simulink model "DoublePendulum"  (R2015a)
settings: Solver=ode45  StartTime=0.0  StopTime=10  RelTol=1e-3
values from neighbouring files (symbols this model uses):
  g = 9.8    [DoublePendulum_config.m]
  J1 = 1.0    (= 1)    [DoublePendulum_config.m]
  J2 = 1.0    (= 1)    [DoublePendulum_config.m]
  l1 = 2.0    (= 2)    [DoublePendulum_config.m]
  l2 = 1.0    (= 1)    [DoublePendulum_config.m]
  lg1 = 1.2    [DoublePendulum_config.m]
  lg2 = 0.5    [DoublePendulum_config.m]
  m1 = 1.0    (= 1)    [DoublePendulum_config.m]
  m2 = 1.0    (= 1)    [DoublePendulum_config.m]
settings Model: Creator=hamada  LastModifiedBy=hamada

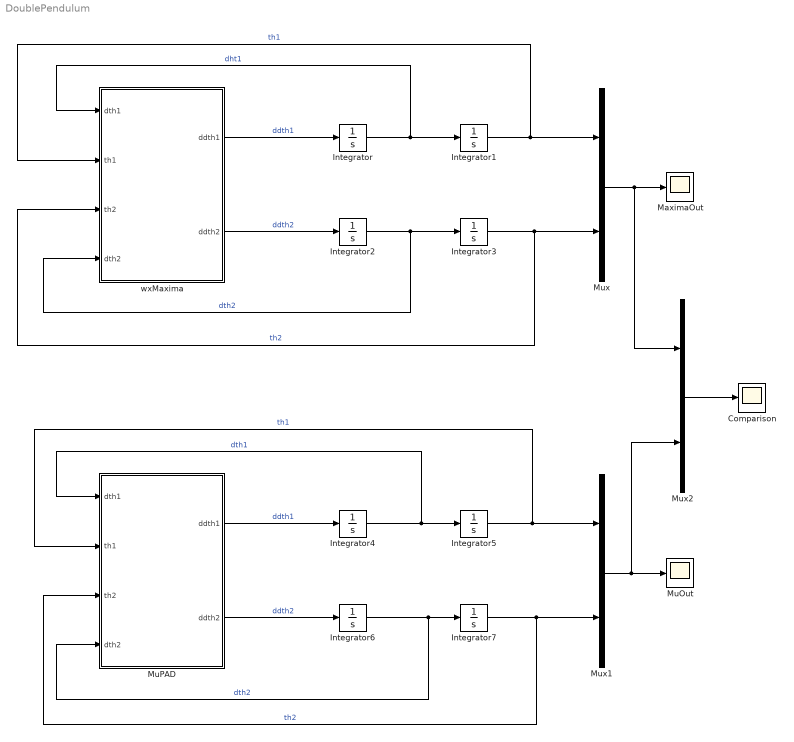
== system DoublePendulum ==
  Comparison : Scope
      settings: TimeRange=10  YMax=15  SaveName=MaximaOut1  SampleInput=on  SampleTime=0.1
  Integrator{,2..4,6..7} (6 alike) : Integrator
  Integrator1 : Integrator  InitialCondition=pi/2
  Integrator5 : Integrator  InitialCondition=pi/2
  MaximaOut : Scope
      settings: TimeRange=10  YMax=15  SaveName=MaximaOut  SampleInput=on  SampleTime=0.1
  MuOut : Scope
      settings: SaveName=MuOut  SampleInput=on  SampleTime=0.1
  MuPAD : MATLAB Function  TreatAsAtomicUnit=on
  Mux : Mux  Inputs=2
  Mux1 : Mux  Inputs=2
  Mux2 : Mux  Inputs=2
  wxMaxima : MATLAB Function  TreatAsAtomicUnit=on
  wires:
  wxMaxima/1(ddth1) -> Integrator/1  "ddth1"
  Integrator/1 -> wxMaxima/1(dth1), Integrator1/1  "dht1"
  Integrator1/1 -> Mux/1, wxMaxima/2(th1)  "th1"
  wxMaxima/2(ddth2) -> Integrator2/1  "ddth2"
  Integrator2/1 -> wxMaxima/4(dth2), Integrator3/1  "dth2"
  Integrator3/1 -> Mux/2, wxMaxima/3(th2)  "th2"
  Mux/1 -> Mux2/1, MaximaOut/1
  MuPAD/1(ddth1) -> Integrator4/1  "ddth1"
  MuPAD/2(ddth2) -> Integrator6/1  "ddth2"
  Integrator4/1 -> MuPAD/1(dth1), Integrator5/1  "dth1"
  Integrator6/1 -> MuPAD/4(dth2), Integrator7/1  "dth2"
  Integrator5/1 -> Mux1/1, MuPAD/2(th1)  "th1"
  Integrator7/1 -> Mux1/2, MuPAD/3(th2)  "th2"
  Mux1/1 -> Mux2/2, MuOut/1
  Mux2/1 -> Comparison/1

== matlab function DoublePendulum/MuPAD ==
  data: dth1 input double size=1; ddth1 output double size=1; th1 input double size=1; th2 input double size=1; dth2 input double size=1; lg1 parameter double size=1; l1 parameter double size=1; lg2 parameter double size=1; l2 parameter double size=1; m1 parameter double size=1; m2 parameter double size=1; J1 parameter double size=1; J2 parameter double size=1; ddth2 output double size=1; g parameter double size=1
function [ ddth1, ddth2 ] = fcn( dth1, th1, th2, dth2, lg1, l1, lg2, l2, m1, m2, J1, J2, g )
    %#codegen
    ddth1 = (sin(th2*2.0)*dth1^2*l1^2*lg2^2*m2^2+g*sin(th1)*l1*lg2^2*m2^2-g*sin(th1+th2*2.0)*l1*lg2^2*m2^2+sin(th2)*dth1^2*l1*lg2^3*m2^2*2.0+sin(th2)*dth2^2*l1*lg2^3*m2^2*2.0+g*sin(th1)*J2*l1*m2*2.0+g*sin(th1)*J2*lg1*m1*2.0+g*sin(th1)*lg1*lg2^2*m1*m2*2.0+sin(th2)*dth1*dth2*l1*lg2^3*m2^2*4.0+sin(th2)*dth1^2*J2*l1*lg2*m2*2.0+sin(th2)*dth2^2*J2*l1*lg2*m2*2.0+sin(th2)*dth1*dth2*J2*l1*lg2*m2*4.0)/(J1*J2*2.0+J2*l1^2*m2*2.0+J2*lg1^2*m1*2.0+J1*lg2^2*m2*2.0+l1^2*lg2^2*m2^2+lg1^2*lg2^2*m1*m2*2.0-cos(th2*2.0)*l1^2*lg2^2*m2^2);
    ddth2 = -(-g*sin(th1+th2)*l1^2*lg2*m2^2-g*sin(th1+th2)*J1*lg2*m2+sin(th2*2.0)*dth1^2*l1^2*lg2^2*m2^2+sin(th2*2.0)*dth2^2*l1^2*lg2^2*m2^2*(1.0/2.0)+g*sin(th1)*l1*lg2^2*m2^2+sin(th2)*dth1^2*l1^3*lg2*m2^2+sin(th2)*dth1^2*l1*lg2^3*m2^2+sin(th2)*dth2^2*l1*lg2^3*m2^2+g*sin(th1)*J2*l1*m2+g*sin(th1)*J2*lg1*m1+g*sin(th1)*lg1*lg2^2*m1*m2+sin(th2*2.0)*dth1*dth2*l1^2*lg2^2*m2^2+g*cos(th2)*sin(th1)*l1^2*lg2*m2^2+sin(th2)*dth1*dth2*l1*lg2^3*m2^2*2.0+sin(th2)*dth1^2*J1*l1*lg2*m2+sin(th2)*dth1^2*J2*l1*lg2*m2+sin(th2)*dth2^2*J2*l1*lg2*m2-g*sin(th1+th2)*lg1^2*lg2*m1*m2-g*sin(th1+th2)*cos(th2)*l1*lg2^2*m2^2+sin(th2)*dth1*dth2*J2*l1*lg2*m2*2.0+sin(th2)*dth1^2*l1*lg1^2*lg2*m1*m2+g*cos(th2)*sin(th1)*l1*lg1*lg2*m1*m2)/(J1*J2+J2*l1^2*m2+J2*lg1^2*m1+J1*lg2^2*m2+l1^2*lg2^2*m2^2+lg1^2*lg2^2*m1*m2-cos(th2)^2*l1^2*lg2^2*m2^2);
end

== matlab function DoublePendulum/wxMaxima ==
  data: dth1 input double size=1; ddth1 output double size=1; th1 input double size=1; th2 input double size=1; dth2 input double size=1; lg1 parameter double size=1; l1 parameter double size=1; lg2 parameter double size=1; l2 parameter double size=1; m1 parameter double size=1; m2 parameter double size=1; J1 parameter double size=1; J2 parameter double size=1; ddth2 output double size=1; g parameter double size=1
function [ ddth1, ddth2 ] = fcn( dth1, th1, th2, dth2, lg1, l1, lg2, l2, m1, m2, J1, J2, g )
    %#codegen
    ddth1 = (g*l1*lg2^2*m2^2*cos(th2)*sin(th2+th1)+(-l1*lg2^3*m2^2-J2*l1*lg2*m2)*sin(th2)*(dth2)^2+(-2*l1*lg2^3*m2^2-2*J2*l1*lg2*m2)*(dth1)*sin(th2)*(dth2)+((-l1*lg2^3*m2^2-J2*l1*lg2*m2)*(dth1)^2-l1^2*lg2^2*m2^2*(dth1)^2*cos(th2))*sin(th2)+(-g*l1*lg2^2*m2^2+(-g*lg1*lg2^2*m1-J2*g*l1)*m2-J2*g*lg1*m1)*sin(th1))/(l1^2*lg2^2*m2^2*cos(th2)^2-l1^2*lg2^2*m2^2+(-lg1^2*lg2^2*m1-J1*lg2^2-J2*l1^2)*m2-J2*lg1^2*m1-J1*J2);
    ddth2 = -((g*l1*lg2^2*m2^2*cos(th2)+g*l1^2*lg2*m2^2+(g*lg1^2*lg2*m1+J1*g*lg2)*m2)*sin(th2+th1)+(-l1^2*lg2^2*m2^2*cos(th2)-l1*lg2^3*m2^2-J2*l1*lg2*m2)*sin(th2)*(dth2)^2+((-2*l1*lg2^3*m2^2-2*J2*l1*lg2*m2)*(dth1)-2*l1^2*lg2^2*m2^2*(dth1)*cos(th2))*sin(th2)*(dth2)+(((-l1*lg2^3-l1^3*lg2)*m2^2+((-J2-J1)*l1*lg2-l1*lg1^2*lg2*m1)*m2)*(dth1)^2-2*l1^2*lg2^2*m2^2*(dth1)^2*cos(th2))*sin(th2)+(-g*l1^2*lg2*m2^2-g*l1*lg1*lg2*m1*m2)*sin(th1)*cos(th2)+(-g*l1*lg2^2*m2^2+(-g*lg1*lg2^2*m1-J2*g*l1)*m2-J2*g*lg1*m1)*sin(th1))/(l1^2*lg2^2*m2^2*cos(th2)^2-l1^2*lg2^2*m2^2+(-lg1^2*lg2^2*m1-J1*lg2^2-J2*l1^2)*m2-J2*lg1^2*m1-J1*J2);
end
